simulink model "MWP_Control"  (Simulink 10.0)
settings: Solver=ode4  StartTime=0.0  StopTime=100  FixedStep=Ts  RelTol=1e-3
values from neighbouring files (symbols this model uses):
  b = 34.5*cm_unit    (= 0.345)    [Parameters.m]
  kv = -2.68    [AssignmentCode.m]
  r0_init = 0    [Initial_Posture.m]
  rw = 7.75*cm_unit    (= 0.0775)    [Parameters.m]
  rx_init = r_init(1)    [Initial_Posture.m]
  ry_init = r_init(2)    [Initial_Posture.m]
  rz_init = r_init(3)    [Initial_Posture.m]
  tauv = 0.05    [AssignmentCode.m]
  theta13_init = 0    [Initial_Posture.m]
  theta13d_init = 0    [Initial_Posture.m]
  theta23_init = 0    [Initial_Posture.m]
  theta23d_init = 0    [Initial_Posture.m]
  v0 = 0.2    [AssignmentCode.m]
  w3l_init = 0    [Initial_Posture.m]
  xCo_init = 0.5    [Initial_Posture.m]
  yCo_init = 0.5    [Initial_Posture.m]
  zCo_init = rw    [Initial_Posture.m]
libraries: simulink x4
settings Model: Creator=kerrm  LastModifiedBy=kerrm
settings DataIOCC: SignalLoggingName=sigsOut
settings OptimizationCC: InitFltsAndDblsToZero=on
settings DebuggingCC: SaveWithParameterizedLinksMsg=none  SignalResolutionControl=TryResolveAllWithWarning  MultiTaskDSMMsg=warning  MultiTaskCondExecSysMsg=none  FcnCallInpInsideContextMsg=warning
settings HardwareCC: TargetUnknown=on
settings SFSimCC: SimUseLocalCustomCode=on  CustomCodeUndefinedFunction=FilterOut
settings RTWCC: RTWUseLocalCustomCode=on
settings GRTTargetCC: TargetFcnLib=ansi_tfl_tmw.mat

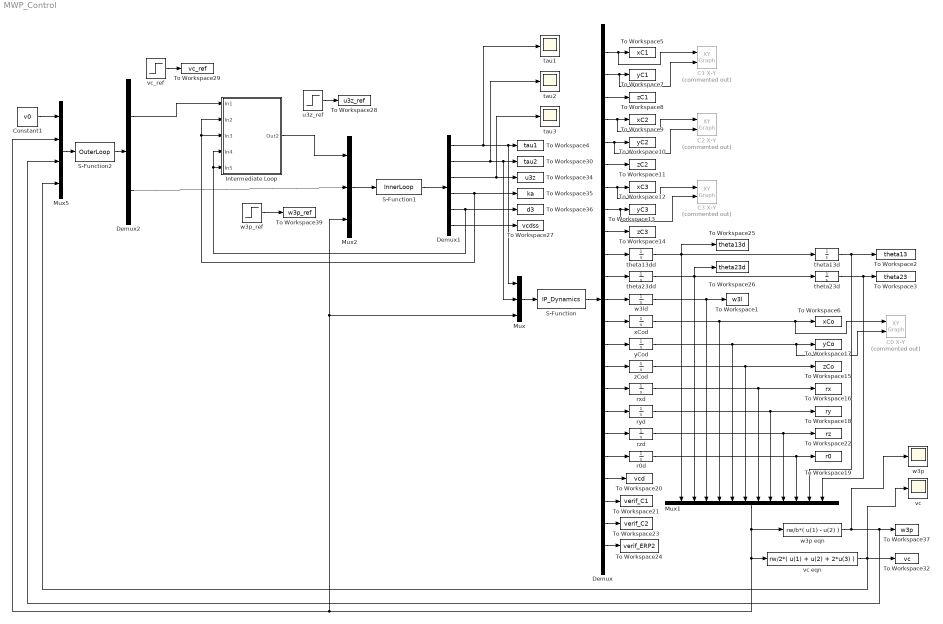
== system MWP_Control ==
  "C0 X-Y " : simulink/Sinks/XY Graph  Commented=on  xmin=0.2  xmax=1.8  ymin=0.2  ymax=1.8  st=-1
  C1 X-Y : simulink/Sinks/XY Graph  Commented=on  xmin=0.2  xmax=1.8  ymin=0.2  ymax=1.8  st=-1
  C2 X-Y : simulink/Sinks/XY Graph  Commented=on  xmin=0.2  xmax=1.8  ymin=0.2  ymax=1.8  st=-1
  C3 X-Y : simulink/Sinks/XY Graph  Commented=on  xmin=0.2  xmax=1.8  ymin=0.2  ymax=1.8  st=-1
  Constant1 : Constant  Value=v0
  Demux : Demux  Outputs=23
  Demux1 : Demux  Outputs=6
  Demux2 : Demux  Outputs=2
  Intermediate Loop : Subsystem
  Mux : Mux  Inputs=3
  Mux1 : Mux  Inputs=12
  Mux2 : Mux  Inputs=3
  Mux5 : Mux
  S-Function : S-Function  FunctionName=IP_Dynamics  SFunctionDeploymentMode=off  EnableBusSupport=off
  S-Function1 : S-Function  FunctionName=InnerLoop  SFunctionDeploymentMode=off  EnableBusSupport=off
  S-Function2 : S-Function  FunctionName=OuterLoop  SFunctionDeploymentMode=off  EnableBusSupport=off
  To Workspace1 : ToWorkspace  VariableName=w3l  SampleTime=-1
  To Workspace10 : ToWorkspace  VariableName=yC2  SampleTime=-1
  To Workspace11 : ToWorkspace  VariableName=zC2  SampleTime=-1
  To Workspace12 : ToWorkspace  VariableName=xC3  SampleTime=-1
  To Workspace13 : ToWorkspace  VariableName=yC3  SampleTime=-1
  To Workspace14 : ToWorkspace  VariableName=zC3  SampleTime=-1
  To Workspace15 : ToWorkspace  VariableName=zCo  SampleTime=-1
  To Workspace16 : ToWorkspace  VariableName=rx  SampleTime=-1
  To Workspace17 : ToWorkspace  VariableName=yCo  SampleTime=-1
  To Workspace18 : ToWorkspace  VariableName=ry  SampleTime=-1
  To Workspace19 : ToWorkspace  VariableName=r0  SampleTime=-1
  To Workspace2 : ToWorkspace  VariableName=theta13  SampleTime=-1
  To Workspace20 : ToWorkspace  VariableName=vcd  SampleTime=-1
  To Workspace21 : ToWorkspace  VariableName=verif_C1  SampleTime=-1
  To Workspace22 : ToWorkspace  VariableName=rz  SampleTime=-1
  To Workspace23 : ToWorkspace  VariableName=verif_C2  SampleTime=-1
  To Workspace24 : ToWorkspace  VariableName=verif_ERP2  SampleTime=-1
  To Workspace25 : ToWorkspace  VariableName=theta13d  SampleTime=-1
  To Workspace26 : ToWorkspace  VariableName=theta23d  SampleTime=-1
  To Workspace27 : ToWorkspace  VariableName=vcdss  SampleTime=-1
  To Workspace28 : ToWorkspace  VariableName=u3z_ref  SampleTime=-1
  To Workspace29 : ToWorkspace  VariableName=vc_ref  SampleTime=-1
  To Workspace3 : ToWorkspace  VariableName=theta23  SampleTime=-1
  To Workspace30 : ToWorkspace  VariableName=tau2  SampleTime=-1
  To Workspace32 : ToWorkspace  VariableName=vc  SampleTime=-1
  To Workspace34 : ToWorkspace  VariableName=u3z  SampleTime=-1
  To Workspace35 : ToWorkspace  VariableName=ka  SampleTime=-1
  To Workspace36 : ToWorkspace  VariableName=d3  SampleTime=-1
  To Workspace37 : ToWorkspace  VariableName=w3p  SampleTime=-1
  To Workspace39 : ToWorkspace  VariableName=w3p_ref  SampleTime=-1
  To Workspace4 : ToWorkspace  VariableName=tau1  SampleTime=-1
  To Workspace5 : ToWorkspace  VariableName=xC1  SampleTime=-1
  To Workspace6 : ToWorkspace  VariableName=xCo  SampleTime=-1
  To Workspace7 : ToWorkspace  VariableName=yC1  SampleTime=-1
  To Workspace8 : ToWorkspace  VariableName=zC1  SampleTime=-1
  To Workspace9 : ToWorkspace  VariableName=xC2  SampleTime=-1
  r0d : Integrator  InitialCondition=r0_init
  rxd : Integrator  InitialCondition=rx_init
  ryd : Integrator  InitialCondition=ry_init
  rzd : Integrator  InitialCondition=rz_init
  tau1 : Scope
  tau2 : Scope
  tau3 : Scope
  theta13d : Integrator  InitialCondition=theta13_init
  theta13dd : Integrator  InitialCondition=theta13d_init
  theta23d : Integrator  InitialCondition=theta23_init
  theta23dd : Integrator  InitialCondition=theta23d_init
  u3z_ref : Step  Time=0  After=0.2  SampleTime=0
  "vc " : Scope
  vc eqn : Fcn  Expr=rw/2*( u(1) + u(2) + 2*u(3) )
  vc_ref : Step  Time=0  After=0.2  SampleTime=0
  w3ld : Integrator  InitialCondition=w3l_init
  w3p : Scope
  "w3p eqn " : Fcn  Expr=rw/b*( u(1) - u(2) )
  w3p_ref : Step  Time=0  SampleTime=0
  xCod : Integrator  InitialCondition=xCo_init
  yCod : Integrator  InitialCondition=yCo_init
  zCod : Integrator  InitialCondition=zCo_init
  wires:
  S-Function/1 -> Demux/1
  zCod/1 -> To Workspace15/1, Mux1/6
  Demux/1 -> C1 X-Y/1, To Workspace5/1
  Demux/2 -> C1 X-Y/2, To Workspace7/1
  Demux/3 -> To Workspace8/1
  Demux/4 -> C2 X-Y/1, To Workspace9/1
  Demux/5 -> C2 X-Y/2, To Workspace10/1
  Demux/6 -> To Workspace11/1
  Demux/7 -> C3 X-Y/1, To Workspace12/1
  Demux/8 -> C3 X-Y/2, To Workspace13/1
  Demux/9 -> To Workspace14/1
  theta13d/1 -> To Workspace2/1, Mux1/11
  theta13dd/1 -> Mux1/1, To Workspace25/1, theta13d/1
  theta23d/1 -> To Workspace3/1, Mux1/12
  theta23dd/1 -> theta23d/1, Mux1/2, To Workspace26/1
  w3ld/1 -> Mux1/3, To Workspace1/1
  r0d/1 -> To Workspace19/1, Mux1/10
  rzd/1 -> To Workspace22/1, Mux1/9
  Mux/1 -> S-Function/1
  xCod/1 -> "C0 X-Y "/1, To Workspace6/1, Mux1/4
  yCod/1 -> "C0 X-Y "/2, To Workspace17/1, Mux1/5
  rxd/1 -> To Workspace16/1, Mux1/7
  ryd/1 -> To Workspace18/1, Mux1/8
  Demux/10 -> theta13dd/1
  Demux/12 -> w3ld/1
  Demux/13 -> xCod/1
  Demux/14 -> yCod/1
  Demux/15 -> zCod/1
  Demux/16 -> rxd/1
  Demux/17 -> ryd/1
  Demux/19 -> r0d/1
  Demux/20 -> To Workspace20/1
  Demux/21 -> To Workspace21/1
  Demux/22 -> To Workspace23/1
  Demux/23 -> To Workspace24/1
  S-Function1/1 -> Demux1/1
  Mux2/1 -> S-Function1/1
  Demux1/1 -> tau1/1, To Workspace4/1, Mux/1
  vc eqn/1 -> Mux5/4, "vc "/1, To Workspace32/1
  Demux1/2 -> tau2/1, Mux/2, To Workspace30/1
  Demux1/3 -> tau3/1, To Workspace34/1
  Demux1/4 -> To Workspace35/1, Intermediate Loop/2(In2), Intermediate Loop/3(In3)
  "w3p eqn "/1 -> Mux5/3, To Workspace37/1, w3p/1
  Demux1/6 -> To Workspace27/1
  Demux/11 -> theta23dd/1
  Demux/18 -> rzd/1
  Mux1/1 -> "w3p eqn "/1, Mux2/3, Mux/3, Mux5/2, vc eqn/1
  Constant1/1 -> Mux5/1
  Demux1/5 -> Intermediate Loop/5(In5), Intermediate Loop/4(In4), To Workspace36/1
  Mux5/1 -> S-Function2/1
  S-Function2/1 -> Demux2/1
  Demux2/2 -> Mux2/2
  vc_ref/1 -> To Workspace29/1
  Demux2/1 -> Intermediate Loop/1(In1)
  Intermediate Loop/1(Out2) -> Mux2/1
  w3p_ref/1 -> To Workspace39/1
  u3z_ref/1 -> To Workspace28/1

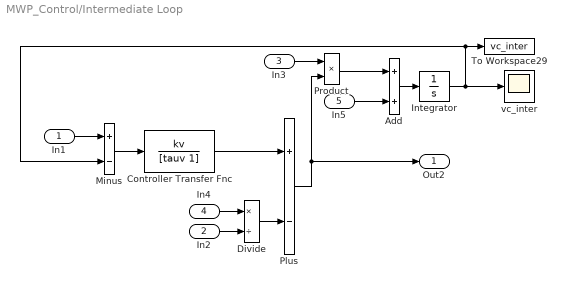
== system MWP_Control/Intermediate Loop ==
  In1 : Inport
  In2 : Inport  Port=2
  In3 : Inport  Port=3
  In4 : Inport  Port=4
  In5 : Inport  Port=5
  Add : Sum
  Controller Transfer Fnc : TransferFcn  Numerator=kv  Denominator=[tauv 1]
  Divide : Product  Inputs=*/
  Integrator : Integrator
  Minus : Sum  Inputs=+-
  Plus : Sum  Inputs=+-
  Product : Product
  To Workspace29 : ToWorkspace  VariableName=vc_inter  SampleTime=-1
  "vc_inter " : Scope
  Out2 : Outport
  wires:
  Divide/1 -> Plus/2
  Minus/1 -> Controller Transfer Fnc/1
  Plus/1 -> Product/2, Out2/1
  Controller Transfer Fnc/1 -> Plus/1
  In1/1 -> Minus/1
  In3/1 -> Product/1
  In2/1 -> Divide/2
  Add/1 -> Integrator/1
  In4/1 -> Divide/1
  Product/1 -> Add/1
  In5/1 -> Add/2
  Integrator/1 -> Minus/2, To Workspace29/1, "vc_inter "/1
